simulink model "cruise_control"  (R2020b)
settings: Solver=VariableStepAuto  StartTime=0.0  StopTime=10.0  RelTol=1e-3
values from neighbouring files (symbols this model uses):
  b = 50    [Cruise_control_data.mat]
  m = 1000    [Cruise_control_data.mat]
settings Model: Creator=JAGRUTI SHINDE  LastModifiedBy=JAGRUTI SHINDE

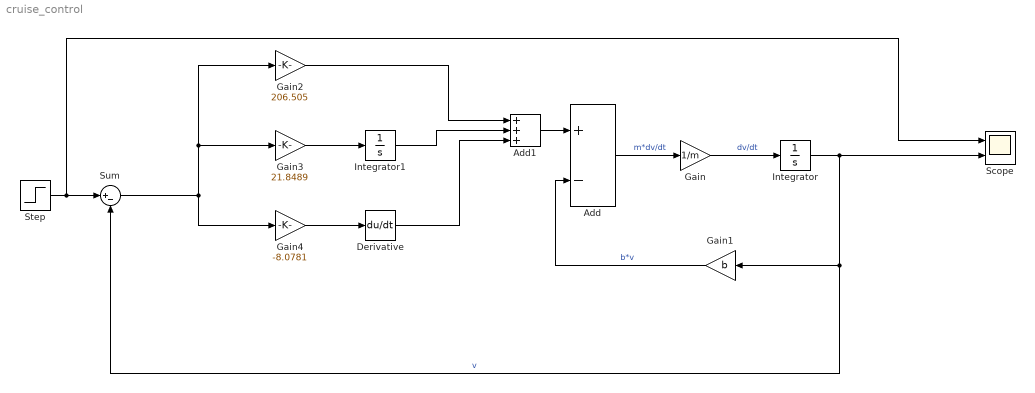
== system cruise_control ==
  Add : Sum  Inputs=+-
  Add1 : Sum  Inputs=+++
  Derivative : Derivative
  Gain : Gain  Gain=1/m
  Gain1 : Gain  Gain=b
  Gain2 : Gain  Gain=206.505
  Gain3 : Gain  Gain=21.8489
  Gain4 : Gain  Gain=-8.0781
  Integrator : Integrator
  Integrator1 : Integrator
  Scope : Scope  NumInputPorts=2
  Step : Step  Time=3  SampleTime=0
  Sum : Sum  Inputs=|+-
  wires:
  Add/1 -> Gain/1  "m*dv/dt"
  Gain/1 -> Integrator/1  "dv/dt"
  Integrator/1 -> Sum/2, Gain1/1, Scope/2  "v"
  Gain1/1 -> Add/2  "b*v"
  Sum/1 -> Gain4/1, Gain3/1, Gain2/1
  Gain3/1 -> Integrator1/1
  Gain4/1 -> Derivative/1
  Gain2/1 -> Add1/1
  Integrator1/1 -> Add1/2
  Derivative/1 -> Add1/3
  Add1/1 -> Add/1
  Step/1 -> Scope/1, Sum/1
